simulink model "MILS_PM"  (R2025b)
settings: Solver=ode4  StartTime=0.0  StopTime=SimEnd  FixedStep=dt  RelTol=1e-3
undefined symbols (not defined in the file): dt, fault_U, fault_V, fault_W, fc, Id_ref, Iq_ref, Ld, Lq, N_rpm, Pp, Psi_a, R, Vdc
libraries: simulink x2
settings Model: Creator=msay5  LastModifiedBy=msay5

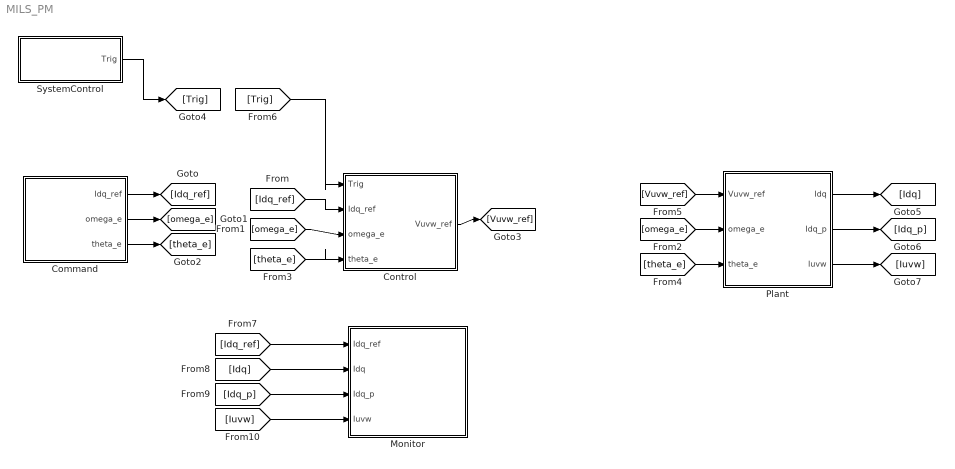
== system MILS_PM ==
  Command : Subsystem
  Control : Subsystem
  Monitor : Subsystem
  Plant : Subsystem
  SystemControl : Subsystem
  wires:
  Control/1(Vuvw_ref) -> [Vuvw_ref]
  SystemControl/1(Trig) -> [Trig]
  Command/1(Idq_ref) -> [Idq_ref]
  [Idq_ref] -> Control/2(Idq_ref)
  Command/2(omega_e) -> [omega_e]
  [omega_e] -> Control/3(omega_e)
  [omega_e] -> Plant/2(omega_e)
  Command/3(theta_e) -> [theta_e]
  [theta_e] -> Control/4(theta_e)
  [theta_e] -> Plant/3(theta_e)
  [Vuvw_ref] -> Plant/1(Vuvw_ref)
  [Trig] -> Control/1(Trig)
  Plant/1(Idq) -> [Idq]
  [Idq_ref] -> Monitor/1(Idq_ref)
  [Idq] -> Monitor/2(Idq)
  Plant/2(Idq_p) -> [Idq_p]
  Plant/3(Iuvw) -> [Iuvw]
  [Idq_p] -> Monitor/3(Idq_p)
  [Iuvw] -> Monitor/4(Iuvw)

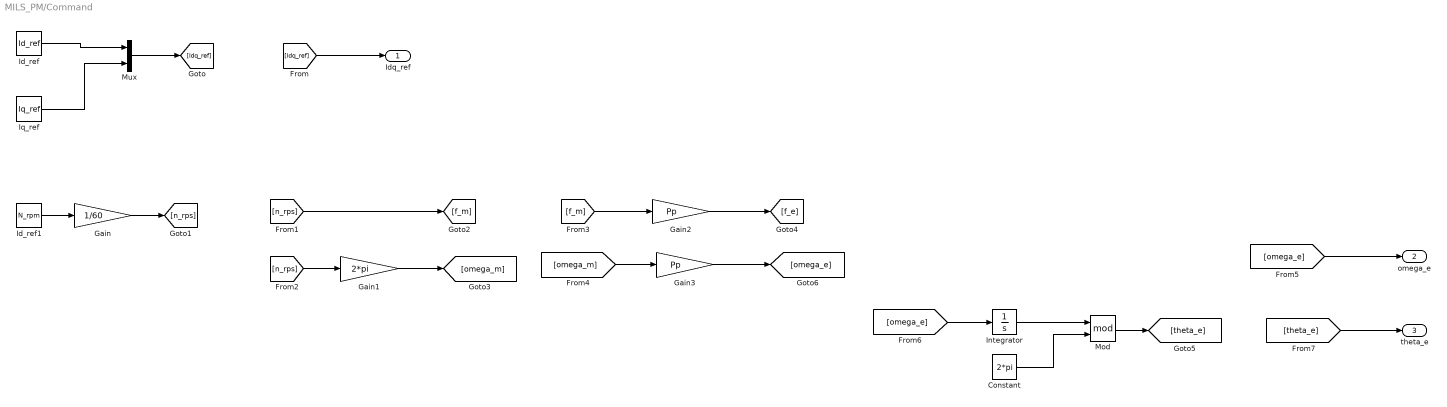
== system MILS_PM/Command ==
  Constant : Constant  Value=2*pi
  Gain : Gain  Gain=1/60
  Gain1 : Gain  Gain=2*pi
  Gain2 : Gain  Gain=Pp
  Gain3 : Gain  Gain=Pp
  Id_ref : Constant  Value=Id_ref
  Id_ref1 : Constant  Value=N_rpm
  Integrator : Integrator
  Iq_ref : Constant  Value=Iq_ref
  Mod : Math  Operator=mod
  Mux : Mux  Inputs=2
  Idq_ref : Outport
  omega_e : Outport  Port=2
  theta_e : Outport  Port=3
  wires:
  Id_ref/1 -> Mux/1
  Iq_ref/1 -> Mux/2
  Mux/1 -> [Idq_ref]
  [Idq_ref] -> Idq_ref/1
  Id_ref1/1 -> Gain/1
  Gain/1 -> [n_rps]
  [n_rps] -> [f_m]
  [n_rps] -> Gain1/1
  Gain1/1 -> [omega_m]
  [f_m] -> Gain2/1
  Gain2/1 -> [f_e]
  [omega_m] -> Gain3/1
  Gain3/1 -> [omega_e]
  [omega_e] -> Integrator/1
  Integrator/1 -> Mod/1
  Constant/1 -> Mod/2
  Mod/1 -> [theta_e]
  [theta_e] -> theta_e/1
  [omega_e] -> omega_e/1

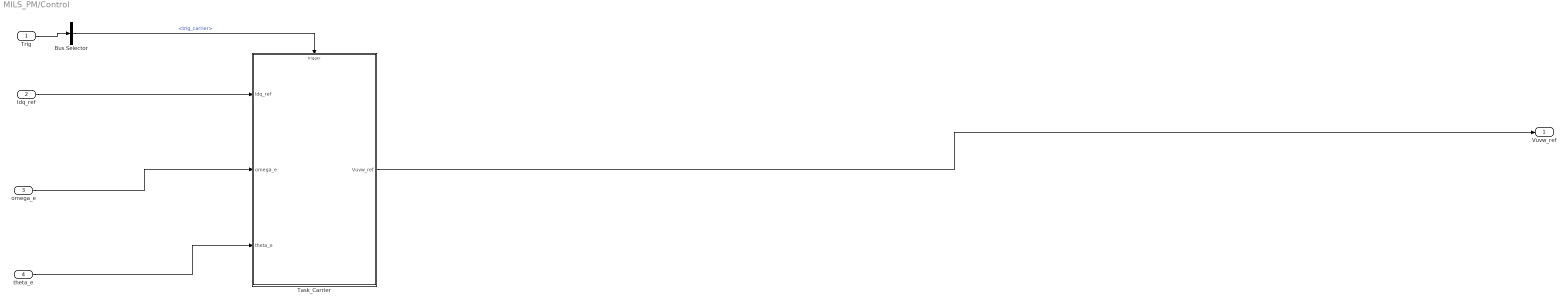
== system MILS_PM/Control ==
  Trig : Inport
  Idq_ref : Inport  Port=2
  omega_e : Inport  Port=3
  theta_e : Inport  Port=4
  Bus Selector : BusSelector  OutputSignals=trig_carrier
  Task_Carrier : Subsystem
  Vuvw_ref : Outport
  wires:
  Idq_ref/1 -> Task_Carrier/1(Idq_ref)
  omega_e/1 -> Task_Carrier/2(omega_e)
  theta_e/1 -> Task_Carrier/3(theta_e)
  Task_Carrier/1(Vuvw_ref) -> Vuvw_ref/1
  Trig/1 -> Bus Selector/1
  Bus Selector/1 -> Task_Carrier/Trigger  "<trig_carrier>"

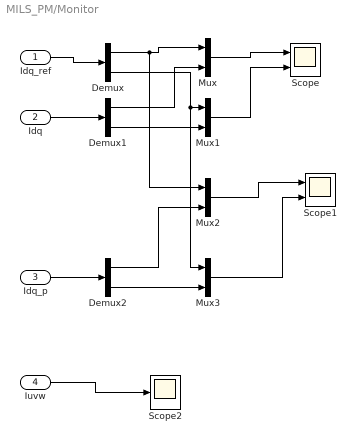
== system MILS_PM/Monitor ==
  Idq_ref : Inport
  Idq : Inport  Port=2
  Idq_p : Inport  Port=3
  Iuvw : Inport  Port=4
  Demux : Demux  Outputs=2
  Demux1 : Demux  Outputs=2
  Demux2 : Demux  Outputs=2
  Mux{,1..3} (4 alike) : Mux  Inputs=2
  Scope : Scope  NumInputPorts=2
      settings: ActiveDisplayYMinimum=-215.14983097456255  ActiveDisplayYMaximum=23.90553677495139  DataLoggingVariableName=ScopeData5
  Scope1 : Scope  NumInputPorts=2
      settings: ActiveDisplayYMinimum=-423.77660834264867  ActiveDisplayYMaximum=420.40069806239126  DataLoggingVariableName=ScopeData6
  Scope2 : Scope
      settings: ActiveDisplayYMinimum=-292.82273187813104  ActiveDisplayYMaximum=292.63981411832225  DataLoggingVariableName=ScopeData7
  wires:
  Idq_ref/1 -> Demux/1
  Idq/1 -> Demux1/1
  Demux/1 -> Mux2/1, Mux/1
  Demux1/1 -> Mux/2
  Demux/2 -> Mux3/1, Mux1/1
  Demux1/2 -> Mux1/2
  Mux1/1 -> Scope/2
  Idq_p/1 -> Demux2/1
  Mux/1 -> Scope/1
  Demux2/1 -> Mux2/2
  Mux2/1 -> Scope1/1
  Demux2/2 -> Mux3/2
  Mux3/1 -> Scope1/2
  Iuvw/1 -> Scope2/1

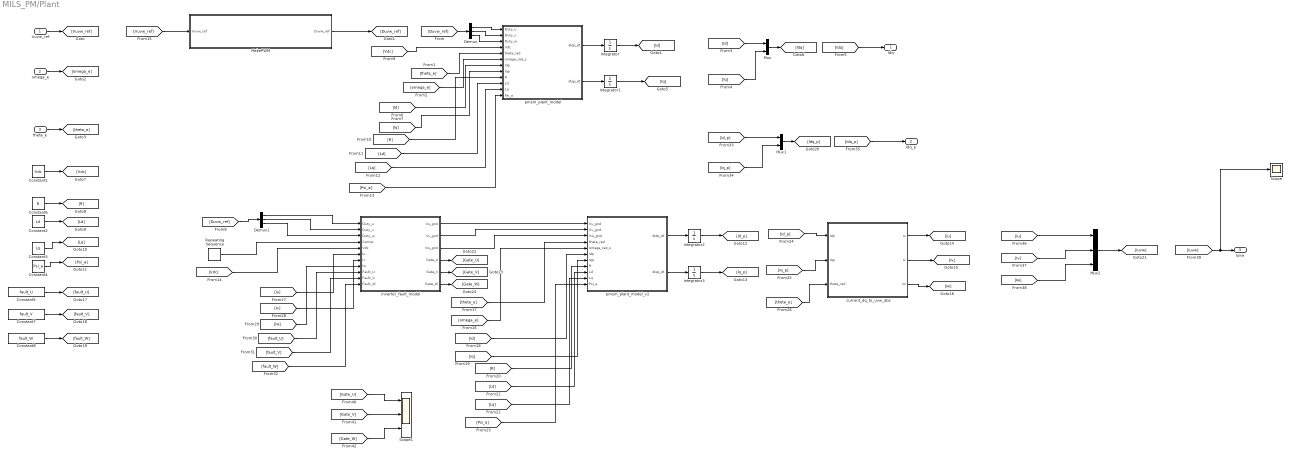
== system MILS_PM/Plant ==
  Vuvw_ref : Inport
  omega_e : Inport  Port=2
  theta_e : Inport  Port=3
  Constant1 : Constant  Value=Vdc
  Constant2 : Constant  Value=Ld
  Constant3 : Constant  Value=Lq
  Constant4 : Constant  Value=Psi_a
  Constant5 : Constant  Value=fault_U
  Constant6 : Constant  Value=R
  Constant7 : Constant  Value=fault_V
  Constant8 : Constant  Value=fault_W
  Demux : Demux  Outputs=3
  Demux1 : Demux  Outputs=3
  Integrator{,1..3} (4 alike) : Integrator
  MakePWM : Subsystem
  Mux : Mux  Inputs=2
  Mux1 : Mux  Inputs=2
  Mux2 : Mux  Inputs=3
  Repeating Sequence : simulink/Sources/Repeating Sequence  rep_seq_t=[0 1/(2*fc) 1/fc]  rep_seq_y=[1 0 1]
  Scope : Scope
      settings: ActiveDisplayYMinimum=-30.212490302281054  ActiveDisplayYMaximum=30.420863819800076  DataLoggingVariableName=ScopeData8
  Scope1 : Scope  NumInputPorts=3
      settings: ActiveDisplayYMinimum=-0.12499999999999997  ActiveDisplayYMaximum=1.125  DataLoggingVariableName=ScopeData9
  current_dq_to_uvw_abs : MATLAB Function  TreatAsAtomicUnit=on
  inverter_fault_model : MATLAB Function  TreatAsAtomicUnit=on
  pmsm_plant_model : MATLAB Function  TreatAsAtomicUnit=on
  pmsm_plant_model_v2 : MATLAB Function  TreatAsAtomicUnit=on
  Idq : Outport
  Idq_p : Outport  Port=2
  Iuvw : Outport  Port=3
  wires:
  Vuvw_ref/1 -> [Vuvw_ref]
  [Vuvw_ref] -> MakePWM/1(Vuvw_ref)
  MakePWM/1(Duvw_ref) -> [Duvw_ref]
  [Duvw_ref] -> Demux/1
  Demux/1 -> pmsm_plant_model/1(Duty_u)
  Demux/2 -> pmsm_plant_model/2(Duty_v)
  Demux/3 -> pmsm_plant_model/3(Duty_w)
  [Vdc] -> pmsm_plant_model/4(Vdc)
  omega_e/1 -> [omega_e]
  theta_e/1 -> [theta_e]
  [theta_e] -> pmsm_plant_model/5(theta_rad)
  [omega_e] -> pmsm_plant_model/6(omega_rad_s)
  pmsm_plant_model/1(dIdp_dt) -> Integrator/1
  pmsm_plant_model/2(dIqp_dt) -> Integrator1/1
  [Id] -> Mux/1
  [Iq] -> Mux/2
  Mux/1 -> [Idq]
  [Idq] -> Idq/1
  [R] -> pmsm_plant_model/9(R)
  [Ld] -> pmsm_plant_model/10(Ld)
  [Lq] -> pmsm_plant_model/11(Lq)
  [Psi_a] -> pmsm_plant_model/12(Psi_a)
  Integrator/1 -> [Id]
  Integrator1/1 -> [Iq]
  [Id] -> pmsm_plant_model/7(Idp)
  [Iq] -> pmsm_plant_model/8(Iqp)
  inverter_fault_model/1(Vu_gnd) -> pmsm_plant_model_v2/1(Vu_gnd)
  inverter_fault_model/2(Vv_gnd) -> pmsm_plant_model_v2/2(Vv_gnd)
  inverter_fault_model/3(Vw_gnd) -> pmsm_plant_model_v2/3(Vw_gnd)
  [Duvw_ref] -> Demux1/1
  Demux1/1 -> inverter_fault_model/1(Duty_u)
  Demux1/2 -> inverter_fault_model/2(Duty_v)
  Demux1/3 -> inverter_fault_model/3(Duty_w)
  Constant1/1 -> [Vdc]
  Constant6/1 -> [R]
  Constant2/1 -> [Ld]
  Constant3/1 -> [Lq]
  Constant4/1 -> [Psi_a]
  Repeating Sequence/1 -> inverter_fault_model/4(Carrier)
  [Vdc] -> inverter_fault_model/5(Vdc)
  [theta_e] -> pmsm_plant_model_v2/4(theta_rad)
  [omega_e] -> pmsm_plant_model_v2/5(omega_rad_s)
  [Id] -> pmsm_plant_model_v2/6(Idp)
  [Iq] -> pmsm_plant_model_v2/7(Iqp)
  [R] -> pmsm_plant_model_v2/8(R)
  [Ld] -> pmsm_plant_model_v2/9(Ld)
  [Lq] -> pmsm_plant_model_v2/10(Lq)
  [Psi_a] -> pmsm_plant_model_v2/11(Psi_a)
  pmsm_plant_model_v2/1(dIdp_dt) -> Integrator2/1
  pmsm_plant_model_v2/2(dIqp_dt) -> Integrator3/1
  Integrator2/1 -> [Id_p]
  Integrator3/1 -> [Iq_p]
  [Id_p] -> current_dq_to_uvw_abs/1(Idp)
  [Iq_p] -> current_dq_to_uvw_abs/2(Iqp)
  [theta_e] -> current_dq_to_uvw_abs/3(theta_rad)
  current_dq_to_uvw_abs/1(Iu) -> [Iu]
  current_dq_to_uvw_abs/2(Iv) -> [Iv]
  current_dq_to_uvw_abs/3(Iw) -> [Iw]
  [Iu] -> inverter_fault_model/6(Iu)
  [Iv] -> inverter_fault_model/7(Iv)
  [Iw] -> inverter_fault_model/8(Iw)
  Constant5/1 -> [fault_U]
  Constant7/1 -> [fault_V]
  Constant8/1 -> [fault_W]
  [fault_U] -> inverter_fault_model/9(Fault_U)
  [fault_V] -> inverter_fault_model/10(Fault_V)
  [fault_W] -> inverter_fault_model/11(Fault_W)
  Mux1/1 -> [Idq_p]
  [Iq_p] -> Mux1/2
  [Id_p] -> Mux1/1
  [Idq_p] -> Idq_p/1
  [Iu] -> Mux2/1
  [Iv] -> Mux2/2
  [Iw] -> Mux2/3
  Mux2/1 -> [Iuvw]
  [Iuvw] -> Scope/1, Iuvw/1
  inverter_fault_model/4(Gate_U) -> [Gate_U]
  inverter_fault_model/5(Gate_V) -> [Gate_V]
  inverter_fault_model/6(Gate_W) -> [Gate_W]
  [Gate_U] -> Scope1/1
  [Gate_V] -> Scope1/2
  [Gate_W] -> Scope1/3

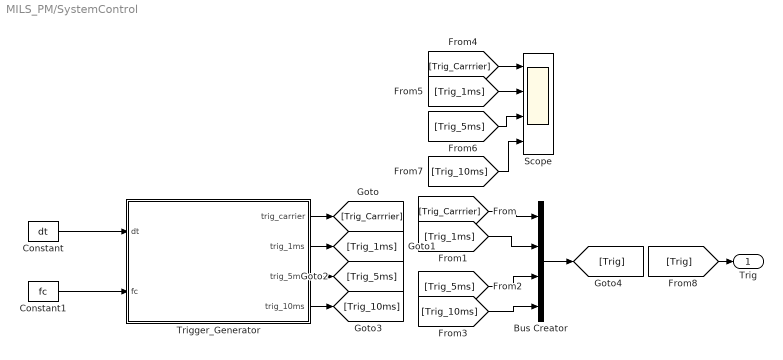
== system MILS_PM/SystemControl ==
  Bus Creator : BusCreator  Inputs=4
  Constant : Constant  Description=基本ステップ時間 dt [s]  Value=dt
      settings: AttributesFormatString=%<Description>
  Constant1 : Constant  Description=キャリア周波数 fc [Hz]  Value=fc
      settings: AttributesFormatString=%<Description>
  Scope : Scope  NumInputPorts=4
      settings: DataLoggingVariableName=ScopeData4
  Trigger_Generator : MATLAB Function  TreatAsAtomicUnit=on
  Trig : Outport
  wires:
  Constant1/1 -> Trigger_Generator/2(fc)
  Bus Creator/1 -> [Trig]
  Trigger_Generator/1(trig_carrier) -> [Trig_Carrrier]
  Constant/1 -> Trigger_Generator/1(dt)
  [Trig_Carrrier] -> Bus Creator/1
  Trigger_Generator/2(trig_1ms) -> [Trig_1ms]
  [Trig_1ms] -> Bus Creator/2
  Trigger_Generator/3(trig_5ms) -> [Trig_5ms]
  [Trig_5ms] -> Bus Creator/3
  Trigger_Generator/4(trig_10ms) -> [Trig_10ms]
  [Trig_10ms] -> Bus Creator/4
  [Trig_Carrrier] -> Scope/1
  [Trig_1ms] -> Scope/2
  [Trig_5ms] -> Scope/3
  [Trig_10ms] -> Scope/4
  [Trig] -> Trig/1

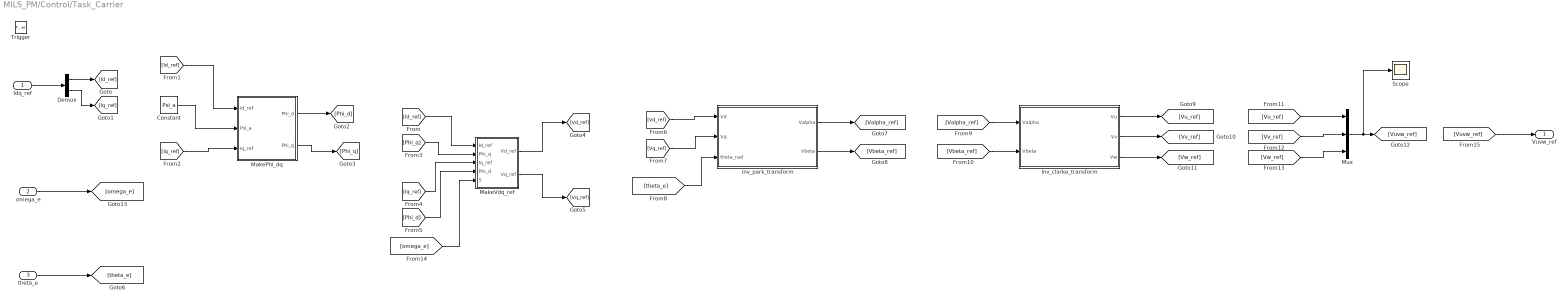
== system MILS_PM/Control/Task_Carrier ==
  Idq_ref : Inport
  omega_e : Inport  Port=2
  theta_e : Inport  Port=3
  Trigger : TriggerPort  VariantControl=(inherit)  PortDimensions=1
  Constant : Constant  Value=Psi_a
  Demux : Demux  Outputs=2
  MakePhi_dq : Subsystem
  MakeVdq_ref : Subsystem
  Mux : Mux  Inputs=3
  Scope : Scope
      settings: ActiveDisplayYMinimum=-255.378930605569  ActiveDisplayYMaximum=255.378930605569
  inv_clarke_transform : MATLAB Function  TreatAsAtomicUnit=on
  inv_park_transform : MATLAB Function  TreatAsAtomicUnit=on
  Vuvw_ref : Outport
  wires:
  Constant/1 -> MakePhi_dq/2(Psi_a)
  Demux/1 -> [Id_ref]
  Demux/2 -> [Iq_ref]
  [Vd_ref] -> inv_park_transform/1(Vd)
  Mux/1 -> Scope/1, [Vuvw_ref]
  [Vuvw_ref] -> Vuvw_ref/1
  [Vw_ref] -> Mux/3
  MakePhi_dq/1(Phi_d) -> [Phi_d]
  [Iq_ref] -> MakeVdq_ref/3(Iq_ref)
  [Iq_ref] -> MakePhi_dq/3(Iq_ref)
  [Valpha_ref] -> inv_clarke_transform/1(Valpha)
  MakePhi_dq/2(Phi_q) -> [Phi_q]
  inv_clarke_transform/1(Vu) -> [Vu_ref]
  [Id_ref] -> MakePhi_dq/1(Id_ref)
  [Phi_d] -> MakeVdq_ref/4(Phi_d)
  MakeVdq_ref/2(Vq_ref) -> [Vq_ref]
  [Vu_ref] -> Mux/1
  [Vv_ref] -> Mux/2
  [Phi_q] -> MakeVdq_ref/2(Phi_q)
  [Id_ref] -> MakeVdq_ref/1(Id_ref)
  [theta_e] -> inv_park_transform/3(theta_rad)
  inv_clarke_transform/2(Vv) -> [Vv_ref]
  MakeVdq_ref/1(Vd_ref) -> [Vd_ref]
  inv_park_transform/1(Valpha) -> [Valpha_ref]
  [Vq_ref] -> inv_park_transform/2(Vq)
  [Vbeta_ref] -> inv_clarke_transform/2(Vbeta)
  inv_park_transform/2(Vbeta) -> [Vbeta_ref]
  Idq_ref/1 -> Demux/1
  theta_e/1 -> [theta_e]
  omega_e/1 -> [omega_e]
  inv_clarke_transform/3(Vw) -> [Vw_ref]
  [omega_e] -> MakeVdq_ref/5(omega_e)

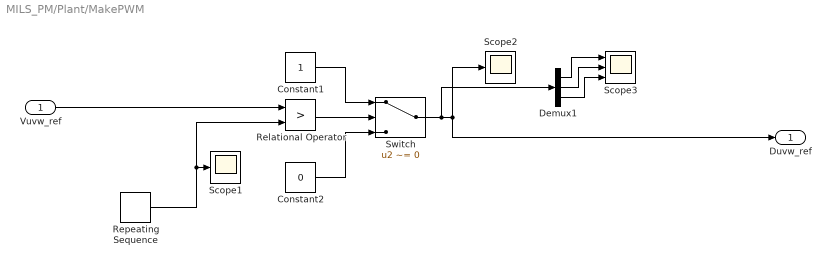
== system MILS_PM/Plant/MakePWM ==
  Vuvw_ref : Inport
  Constant1 : Constant
  Constant2 : Constant  Value=0
  Demux1 : Demux  Outputs=3
  Relational Operator : RelationalOperator  Operator=>  OutDataTypeStr=boolean  RndMeth=Simplest  InputSameDT=off
  Repeating Sequence : simulink/Sources/Repeating Sequence  rep_seq_t=[0 1/(2*fc) 1/fc]  rep_seq_y=[Vdc/2 -Vdc/2 Vdc/2]
  Scope1 : Scope
      settings: ActiveDisplayYMinimum=-150  ActiveDisplayYMaximum=150
  Scope2 : Scope
      settings: ActiveDisplayYMinimum=-33.678550864187159  ActiveDisplayYMaximum=14.887495616436901  DataLoggingVariableName=ScopeData2
  Scope3 : Scope  NumInputPorts=3
      settings: ActiveDisplayYMinimum=-0.12499999999999997  ActiveDisplayYMaximum=1.125  DataLoggingVariableName=ScopeData3
  Switch : Switch  Criteria=u2 ~= 0  SaturateOnIntegerOverflow=off  InputSameDT=off
  Duvw_ref : Outport
  wires:
  Demux1/1 -> Scope3/1
  Switch/1 -> Demux1/1, Duvw_ref/1, Scope2/1
  Demux1/2 -> Scope3/2
  Relational Operator/1 -> Switch/2
  Constant2/1 -> Switch/3
  Demux1/3 -> Scope3/3
  Repeating Sequence/1 -> Relational Operator/2, Scope1/1
  Constant1/1 -> Switch/1
  Vuvw_ref/1 -> Relational Operator/1

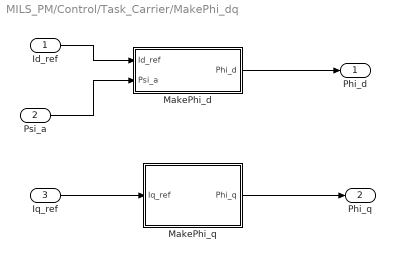
== system MILS_PM/Control/Task_Carrier/MakePhi_dq ==
  Id_ref : Inport
  Psi_a : Inport  Port=2
  Iq_ref : Inport  Port=3
  MakePhi_d : Subsystem
  MakePhi_q : Subsystem
  Phi_d : Outport
  Phi_q : Outport  Port=2
  wires:
  Id_ref/1 -> MakePhi_d/1(Id_ref)
  MakePhi_d/1(Phi_d) -> Phi_d/1
  Psi_a/1 -> MakePhi_d/2(Psi_a)
  MakePhi_q/1(Phi_q) -> Phi_q/1
  Iq_ref/1 -> MakePhi_q/1(Iq_ref)

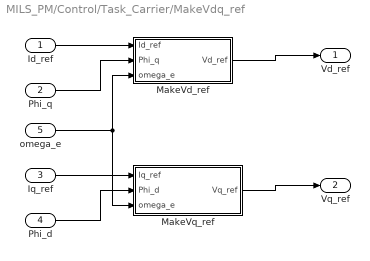
== system MILS_PM/Control/Task_Carrier/MakeVdq_ref ==
  Id_ref : Inport
  Phi_q : Inport  Port=2
  Iq_ref : Inport  Port=3
  Phi_d : Inport  Port=4
  omega_e : Inport  Port=5
  MakeVd_ref : Subsystem
  MakeVq_ref : Subsystem
  Vd_ref : Outport
  Vq_ref : Outport  Port=2
  wires:
  MakeVq_ref/1(Vq_ref) -> Vq_ref/1
  Phi_d/1 -> MakeVq_ref/2(Phi_d)
  Iq_ref/1 -> MakeVq_ref/1(Iq_ref)
  Phi_q/1 -> MakeVd_ref/2(Phi_q)
  Id_ref/1 -> MakeVd_ref/1(Id_ref)
  MakeVd_ref/1(Vd_ref) -> Vd_ref/1
  omega_e/1 -> MakeVq_ref/3(omega_e), MakeVd_ref/3(omega_e)

== system MILS_PM/Control/Task_Carrier/MakePhi_dq/MakePhi_d ==
  Id_ref : Inport
  Psi_a : Inport  Port=2
  Add : Sum
  Gain1 : Gain  Gain=Ld
  Phi_d : Outport
  wires:
  Id_ref/1 -> Gain1/1
  Gain1/1 -> Add/1
  Psi_a/1 -> Add/2
  Add/1 -> Phi_d/1

== system MILS_PM/Control/Task_Carrier/MakePhi_dq/MakePhi_q ==
  Iq_ref : Inport
  Gain1 : Gain  Gain=Lq
  Phi_q : Outport
  wires:
  Iq_ref/1 -> Gain1/1
  Gain1/1 -> Phi_q/1

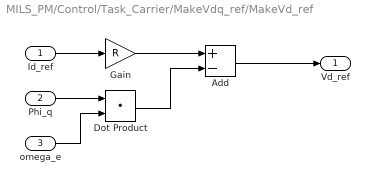
== system MILS_PM/Control/Task_Carrier/MakeVdq_ref/MakeVd_ref ==
  Id_ref : Inport
  Phi_q : Inport  Port=2
  omega_e : Inport  Port=3
  Add : Sum  Inputs=+-
  Dot Product : DotProduct  OutDataTypeStr=Inherit: Inherit via internal rule
  Gain : Gain  Gain=R
  Vd_ref : Outport
  wires:
  Gain/1 -> Add/1
  Phi_q/1 -> Dot Product/1
  Dot Product/1 -> Add/2
  Id_ref/1 -> Gain/1
  Add/1 -> Vd_ref/1
  omega_e/1 -> Dot Product/2

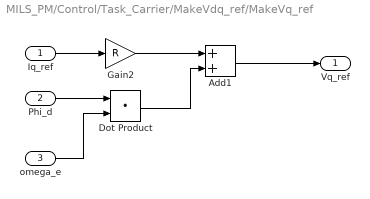
== system MILS_PM/Control/Task_Carrier/MakeVdq_ref/MakeVq_ref ==
  Iq_ref : Inport
  Phi_d : Inport  Port=2
  omega_e : Inport  Port=3
  Add1 : Sum
  Dot Product : DotProduct  OutDataTypeStr=Inherit: Inherit via internal rule
  Gain2 : Gain  Gain=R
  Vq_ref : Outport
  wires:
  Gain2/1 -> Add1/1
  Dot Product/1 -> Add1/2
  Iq_ref/1 -> Gain2/1
  Phi_d/1 -> Dot Product/1
  Add1/1 -> Vq_ref/1
  omega_e/1 -> Dot Product/2

== matlab function MILS_PM/Plant/pmsm_plant_model_v2 ==
  settings: updateMethod=DISCRETE
  data: Vu_gnd input; dIdp_dt output; Vv_gnd input; Vw_gnd input; theta_rad input; omega_rad_s input; Idp input; Iqp input; R input; dIqp_dt output; Ld input; Lq input; Psi_a input
function [dIdp_dt, dIqp_dt] = pmsm_plant_model_abs(Vu_gnd, Vv_gnd, Vw_gnd, theta_rad, omega_rad_s, Idp, Iqp, R, Ld, Lq, Psi_a)
    % =========================================================================
    % 【連続系プラントモデル（絶対値変換 / 電力不変系）】
    % インバータモデルからの対地電圧を受け取り、電流の微分値(di/dt)を計算して
    % 外部の積分器ブロック(1/s)へ渡すためのモータモデルです。
    %
    % Inputs:
    %   Vu_gnd, Vv_gnd, Vw_gnd : インバータが出力する各相の対地電圧（GND基準） [V]
    %   theta_rad              : 現在のロータ電気角 [rad]
    %   omega_rad_s            : 現在のロータ電気角速度 [rad/s]
    %   Idp, Iqp               : 現在のd軸・q軸電流（※絶対値変換スケール） [A]
    %                            <- 外部の積分器からフィードバックされる値
    %   R                      : 巻線抵抗 [Ohm]
    %   Ld, Lq                 : d軸・q軸インダクタンス [H]
    %   Psi_a                  : 永久磁石の鎖交磁束（※物理スケール） [Wb]
    %
    % Outputs:
    %   dIdp_dt, dIqp_dt       : d軸・q軸電流の変化率（※絶対値変換スケール） [A/s]
    %                            -> 外部の積分器(1/s)へ渡す値
    % =========================================================================

    % 定数項の定義（最適化用）
    SQRT_3_2 = sqrt(1.5);
    SQRT_1_2 = sqrt(0.5);

    % --- 1. 中性点電圧の計算と相電圧への変換 ---
    % インバータから直接「対地電圧(V)」を受け取るため、Duty * Vdc の計算は不要です。
    % 3相の対地電圧の平均をとることで、スター結線モータの中性点電圧変動分を算出します。
    Vn_gnd = (Vu_gnd + Vv_gnd + Vw_gnd) / 3.0;
    
    % 対地電圧から中性点電圧を差し引き、モータコイルにかかる真の相電圧を求めます。
    Vu = Vu_gnd - Vn_gnd;
    Vv = Vv_gnd - Vn_gnd;
    Vw = Vw_gnd - Vn_gnd;

    % --- 2. 絶対値Clarke変換（三相物理スケール -> 電力不変α-β） ---
    % 平衡三相(Vu+Vv+Vw=0)を前提に簡略化された絶対値変換式です。
    Valpha_p = SQRT_3_2 * Vu;
    Vbeta_p  = SQRT_1_2 * (Vv - Vw);
    
    % --- 3. Park変換（電力不変α-β -> 電力不変d-q） ---
    cos_th = cos(theta_rad);
    sin_th = sin(theta_rad);
    Vdp = Valpha_p * cos_th + Vbeta_p * sin_th;
    Vqp = -Valpha_p * sin_th + Vbeta_p * cos_th;

    % --- 4. 鎖交磁束の絶対値変換 ---
    % 入力された物理パラメータ Psi_a を電力不変スケールに引き伸ばします。
    Psi_ap = SQRT_3_2 * Psi_a;

    % --- 5. 電圧方程式による電流変化率 (di_p/dt) の計算 ---
    % 外部の積分器からフィードバックされた現在の電流 Idp, Iqp を使用して微分値を算出します。
    dIdp_dt = (Vdp - R * Idp + omega_rad_s * Lq * Iqp) / Ld;
    dIqp_dt = (Vqp - R * Iqp - omega_rad_s * Ld * Idp - omega_rad_s * Psi_ap) / Lq;
end

== matlab function MILS_PM/Plant/current_dq_to_uvw_abs ==
  settings: updateMethod=DISCRETE
  data: Idp input; Iqp input; Iu output; theta_rad input; Iv output; Iw output
function [Iu, Iv, Iw] = current_dq_to_uvw_abs(Idp, Iqp, theta_rad)
    % =========================================================================
    % 【絶対値変換版】d-q軸電流 -> U-V-W相電流 変換モデル
    % 電力不変スケールのIdp, Iqpを、物理スケールの相電流に復元します。
    %
    % Inputs:
    %   Idp, Iqp  : d軸・q軸電流（※絶対値変換スケール） [A]
    %   theta_rad : 現在のロータ電気角 [rad]
    %
    % Outputs:
    %   Iu, Iv, Iw: 物理的な各相電流（インバータモデルの還流判定用） [A]
    % =========================================================================

    % 1. 逆Park変換 (Idp, Iqp -> Ialpha_p, Ibeta_p)
    cos_th = cos(theta_rad);
    sin_th = sin(theta_rad);
    
    Ialpha_p = Idp * cos_th - Iqp * sin_th;
    Ibeta_p  = Idp * sin_th + Iqp * cos_th;

    % 2. 絶対値・逆Clarke変換 (Ialpha_p, Ibeta_p -> Iu, Iv, Iw)
    % 定数項の定義（最適化用）
    % K1 = sqrt(2/3)
    % K2 = -0.5 * sqrt(2/3)
    % K3 = (sqrt(3)/2) * sqrt(2/3) = sqrt(2)/2
    K1 = sqrt(2/3);
    K2 = K1 * -0.5;
    K3 = sqrt(2) / 2;

    Iu = K1 * Ialpha_p;
    Iv = K2 * Ialpha_p + K3 * Ibeta_p;
    Iw = K2 * Ialpha_p - K3 * Ibeta_p;
end

== matlab function MILS_PM/Control/Task_Carrier/inv_clarke_transform ==
  data: Valpha input; Vu output; Vbeta input; Vv output; Vw output
function [Vu, Vv, Vw] = inv_clarke_transform(Valpha, Vbeta)
    % 逆Clarke変換（α-β座標 -> U-V-W座標）
    %
    % Inputs:
    %   Valpha : α軸電圧 [V]
    %   Vbeta  : β軸電圧 [V]
    %
    % Outputs:
    %   Vu     : U相電圧 [V]
    %   Vv     : V相電圧 [V]
    %   Vw     : W相電圧 [V]

    % 定数項の定義（Cコード生成時の最適化用）
    % ※通常コンパイラが定数として解釈しますが、定数であることを明示しています
    SQRT3_OVER_2 = sqrt(3) / 2;

    % 逆Clarke変換の演算
    k = sqrt(2/3);
    Vu = k * Valpha;
    Vv = k * (-0.5 * Valpha + SQRT3_OVER_2 * Vbeta);
    Vw = k * (-0.5 * Valpha - SQRT3_OVER_2 * Vbeta);
end

== matlab function MILS_PM/Control/Task_Carrier/inv_park_transform ==
  data: Vd input; Valpha output; Vq input; theta_rad input; Vbeta output
function [Valpha, Vbeta] = inv_park_transform(Vd, Vq, theta_rad)
    % 逆Park変換（d-q座標 -> α-β座標）
    %
    % Inputs:
    %   Vd        : d軸電圧指令 [V]
    %   Vq        : q軸電圧指令 [V]
    %   theta_rad : モータの電気角 [rad]
    %
    % Outputs:
    %   Valpha    : α軸電圧 [V]
    %   Vbeta     : β軸電圧 [V]

    % Cコード生成時の演算最適化のため、三角関数を一度だけ計算して変数に格納
    cos_th = cos(theta_rad);
    sin_th = sin(theta_rad);

    % 逆Park変換の演算
    Valpha = Vd * cos_th - Vq * sin_th;
    Vbeta  = Vd * sin_th + Vq * cos_th;
end

== matlab function MILS_PM/SystemControl/Trigger_Generator ==
  settings: updateMethod=DISCRETE  sampleTime=dt
  data: dt input; trig_carrier output; fc input; trig_1ms output; trig_5ms output; trig_10ms output
function [trig_carrier, trig_1ms, trig_5ms, trig_10ms] = task_triggers(dt, fc)
    % TASK_TRIGGERS 各周期タスクのトリガ(boolean)を生成する
    %   基本サンプル時間 dt 毎に呼ばれ、カウンタで各周期の立ち上がりを生成する。
    %   ※このブロックのサンプル時間は dt に設定すること。
    %
    % [入力]
    %   dt : 基本サンプル時間 [s]
    %   fc : キャリア周波数 [Hz]
    %
    % [出力]
    %   trig_carrier : キャリア周期トリガ
    %   trig_1ms     : 1ms 周期トリガ
    %   trig_5ms     : 5ms 周期トリガ
    %   trig_10ms    : 10ms 周期トリガ
    %#codegen

    % ==========================================
    % 1. 周期設定
    % ==========================================
    Ts        = dt;       % 基本サンプル時間
    T_carrier = 1 / fc;   % キャリア周期

    % ==========================================
    % 2. カウンタ(永続変数)の初期化
    % ==========================================
    persistent cnt_carrier cnt_1ms cnt_5ms cnt_10ms
    if isempty(cnt_carrier)
        cnt_carrier = uint32(0);
        cnt_1ms     = uint32(0);
        cnt_5ms     = uint32(0);
        cnt_10ms    = uint32(0);
    end

    % ==========================================
    % 3. 各周期の閾値(何ステップでトリガを立てるか)
    % ==========================================
    thresh_carrier = uint32(round(T_carrier / Ts));
    thresh_1ms     = uint32(round(0.001 / Ts));
    thresh_5ms     = uint32(round(0.005 / Ts));
    thresh_10ms    = uint32(round(0.010 / Ts));

    % ==========================================
    % 4. トリガ判定 (閾値到達で true、カウンタリセット)
    % ==========================================
    cnt_carrier = cnt_carrier + 1;
    if cnt_carrier >= thresh_carrier
        trig_carrier = true;
        cnt_carrier  = uint32(0);
    else
        trig_carrier = false;
    end

    cnt_1ms = cnt_1ms + 1;
    if cnt_1ms >= thresh_1ms
        trig_1ms = true;
        cnt_1ms  = uint32(0);
    else
        trig_1ms = false;
    end

    cnt_5ms = cnt_5ms + 1;
    if cnt_5ms >= thresh_5ms
        trig_5ms = true;
        cnt_5ms  = uint32(0);
    else
        trig_5ms = false;
    end

    cnt_10ms = cnt_10ms + 1;
    if cnt_10ms >= thresh_10ms
        trig_10ms = true;
        cnt_10ms  = uint32(0);
    else
        trig_10ms = false;
    end

end

== matlab function MILS_PM/Plant/pmsm_plant_model ==
  settings: updateMethod=DISCRETE
  data: Duty_u input; dIdp_dt output; Duty_v input; Duty_w input; Vdc input; theta_rad input; omega_rad_s input; Idp input; Iqp input; dIqp_dt output; R input; Ld input; Lq input; Psi_a input
function [dIdp_dt, dIqp_dt] = pmsm_plant_model_abs(Duty_u, Duty_v, Duty_w, Vdc, theta_rad, omega_rad_s, Idp, Iqp, R, Ld, Lq, Psi_a)
    % 【連続系プラントモデル（絶対値変換 / 電力不変系）】
    % 電流の微分値 (di_p/dt) を計算し、外部の積分器(1/s)へ渡します。
    
    % 定数項の定義（最適化用）
    SQRT_3_2 = sqrt(1.5);
    SQRT_1_2 = sqrt(0.5);

    % 1. インバータ出力電圧とモータ相電圧の計算（ここは物理スケール）
    Vu_gnd = Duty_u * Vdc;
    Vv_gnd = Duty_v * Vdc;
    Vw_gnd = Duty_w * Vdc;

    % 中性点電圧の計算と相電圧への変換
    Vn_gnd = (Vu_gnd + Vv_gnd + Vw_gnd) / 3.0;
    Vu = Vu_gnd - Vn_gnd;
    Vv = Vv_gnd - Vn_gnd;
    Vw = Vw_gnd - Vn_gnd;

    % 2. 絶対値Clarke変換（三相物理スケール -> 電力不変α-β）
    % 電力不変の変換行列を適用。平衡三相(Vu+Vv+Vw=0)を前提に簡略化しています。
    Valpha_p = SQRT_3_2 * Vu;
    Vbeta_p  = SQRT_1_2 * (Vv - Vw);

    % 3. Park変換（電力不変α-β -> 電力不変d-q）
    cos_th = cos(theta_rad);
    sin_th = sin(theta_rad);
    Vdp = Valpha_p * cos_th + Vbeta_p * sin_th;
    Vqp = -Valpha_p * sin_th + Vbeta_p * cos_th;

    % 4. 鎖交磁束の絶対値変換（★極めて重要）
    % 入力された物理パラメータ Psi_a を電力不変スケールに変換します
    Psi_ap = SQRT_3_2 * Psi_a;

    % 5. 電圧方程式による電流変化率 (di_p/dt) の計算
    % 入力として受け取った電力不変系の Idp, Iqp を使用します
    dIdp_dt = (Vdp - R * Idp + omega_rad_s * Lq * Iqp) / Ld;
    dIqp_dt = (Vqp - R * Iqp - omega_rad_s * Ld * Idp - omega_rad_s * Psi_ap) / Lq;
end

== matlab function MILS_PM/Plant/inverter_fault_model ==
  settings: updateMethod=DISCRETE
  data: Duty_u input; Duty_v input; Duty_w input; Carrier input; Vdc input; Vu_gnd output; Vv_gnd output; Iu input; Iv input; Iw input; Fault_U input; Fault_V input; Fault_W input; Vw_gnd output; Gate_U output; Gate_V output; Gate_W output
function [Vu_gnd, Vv_gnd, Vw_gnd, Gate_U, Gate_V, Gate_W] = ...
    inverter_fault_model(Duty_u, Duty_v, Duty_w, Carrier, Vdc, Iu, Iv, Iw, Fault_U, Fault_V, Fault_W)
    % PWMスイッチング生成およびアーム故障模擬インバータモデル
    %
    % Inputs:
    %   Duty_u, _v, _w : デューティ指令 (0.0 ~ 1.0)
    %   Carrier        : 三角波キャリア信号 (0.0 ~ 1.0) ※外部のRepeating Sequence等で生成
    %   Vdc            : DCリンク電圧 [V]
    %   Iu, Iv, Iw     : モータの各相電流 [A] (還流ダイオードの挙動模擬に必須)
    %   Fault_U, _V, _W: 故障モードフラグ
    %                    0: 正常 (Normal)
    %                    1: 上アーム・オープン故障 (Stuck OFF)
    %                    2: 上アーム・ショート故障 (Stuck ON)
    %                    3: 下アーム・オープン故障 (Stuck OFF)
    %                    4: 下アーム・ショート故障 (Stuck ON)
    %
    % Outputs:
    %   Vu_gnd, _v, _w : 各相の対地電圧 [V] (これをモータモデルの中性点計算へ渡す)
    %   Gate_U, _V, _W : ゲート信号の実際の状態 [上アーム, 下アーム] (1=ON, 0=OFF) デバッグ用

    % 各相の処理を関数化して呼び出し
    [Vu_gnd, Gate_U] = calc_phase_voltage(Duty_u, Carrier, Vdc, Iu, Fault_U);
    [Vv_gnd, Gate_V] = calc_phase_voltage(Duty_v, Carrier, Vdc, Iv, Fault_V);
    [Vw_gnd, Gate_W] = calc_phase_voltage(Duty_w, Carrier, Vdc, Iw, Fault_W);

end

% --- ローカル関数：1相分のゲート信号と出力電圧を計算 ---
function [V_gnd, Gate_State] = calc_phase_voltage(Duty, Carrier, Vdc, I_phase, Fault_Mode)
    
    % 1. 理想的なゲート指令の生成 (デッドタイムは無視)
    % 【修正】比較結果(logical)を double 型(1 または 0) に変換します
    G_up_cmd  = double(Duty >= Carrier);
    G_low_cmd = 1.0 - G_up_cmd;  % 上アームの反転 (1 -> 0, 0 -> 1)

    % 2. 故障の注入 (ゲート実際の状態)
    % 最初から double 型なので、後で 0 や 1 を代入してもエラーになりません
    G_up_act  = G_up_cmd;
    G_low_act = G_low_cmd;
    
    switch Fault_Mode
        case 1 % 上アーム・オープン故障 (常にOFF)
            G_up_act = 0;
        case 2 % 上アーム・ショート故障 (常にON)
            G_up_act = 1;
        case 3 % 下アーム・オープン故障 (常にOFF)
            G_low_act = 0;
        case 4 % 下アーム・ショート故障 (常にON)
            G_low_act = 1;
        otherwise % 0: 正常
            % 何もしない
    end
    
    % 3. スイッチ状態と電流方向に基づく出力電圧の決定
    % （ここから下の if - elseif は前回の修正版のままでOKです）
    if G_up_act == 1 && G_low_act == 0
        % 上のみON -> Vdc出力
        V_gnd = Vdc;
        
    elseif G_up_act == 0 && G_low_act == 1
        % 下のみON -> 0V出力 (GND)
        V_gnd = 0;
        
    elseif G_up_act == 0 && G_low_act == 0
        % 上下OFF (デッドタイム中、またはオープン故障時)
        % 相電流の方向によって還流ダイオードの経路が変わる
        if I_phase > 0
            % モータへ向かって電流が流れている -> 下アームのダイオードを通って還流
            V_gnd = 0;
        else
            % インバータへ向かって電流が戻っている -> 上アームのダイオードを通って還流
            V_gnd = Vdc;
        end
        
    else
        % 短絡 (アームショート・貫通)
        % 実際には素子破壊やヒューズ溶断が起きるが、シミュレーション上は0V(またはVdc/2)とする
        V_gnd = 0; 
    end
    
    % デバッグ出力用
    Gate_State = [G_up_act, G_low_act];
end
